simulink model "Model"  (R2022b)
settings: Solver=FixedStepAuto  StartTime=0.0  StopTime=ts  FixedStep=0.001  RelTol=1e-3
values from neighbouring files (symbols this model uses):
  A1 = 1    [Init.m]    (also in sh.m)
  A2 = 0    [Init.m]    (also in sh.m)
  alpha1 = 0.14    [Init.m]    (also in sh.m)
  alpha2 = 0    [Init.m]    (also in sh.m)
  base = 0.025    [Init.m]
  betta = 0    [Init.m]    (also in sh.m)
  ke = U/w    (= 0.690310596543)    [Init.m]
  km = i*(M/I)    (= 24.1911764706)    [Init.m]
  rad_wheel = 0.02    [Init.m]
  Tm = (J*w)/M0    (= 0.000140723404261)    [Init.m]
  x = 2    [Init.m]
  y = 2    [Init.m]    (also in Shum.m = block1+block2)
undefined symbols (not defined in the file or in its folder): out
libraries: simulink x3, fuzblock x1
settings Model: Creator=Адель  LastModifiedBy=Адель
settings ModelReferenceCC: EnableRefExpFcnMdlSchedulingChecks=on

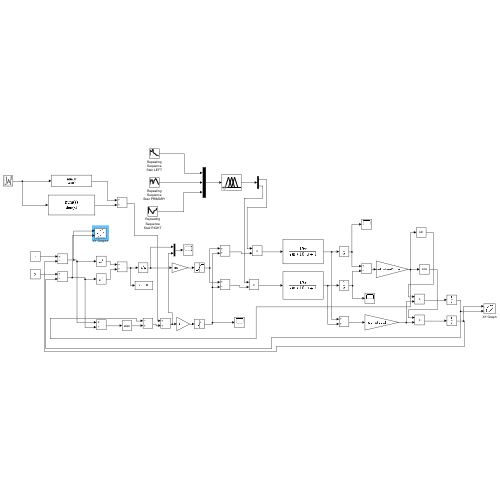
[thumbnail: Simulink's stored preview of the top-level diagram]
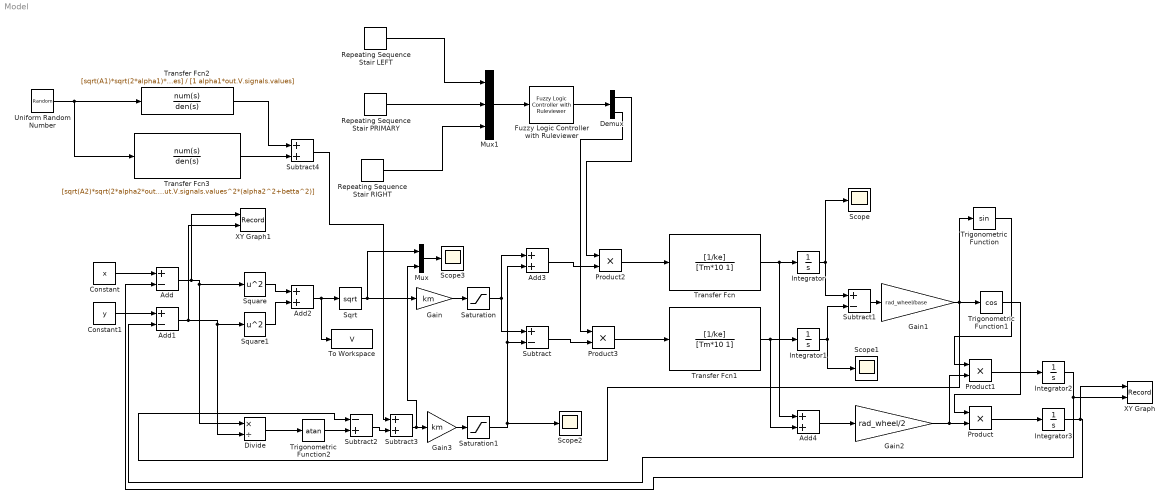
== system Model ==
  Add : Sum  Inputs=+-
  Add1 : Sum  Inputs=+-
  Add2 : Sum
  Add3 : Sum
  Add4 : Sum
  Constant : Constant  Value=x
  Constant1 : Constant  Value=y
  Demux : Demux  Outputs=2
  Divide : Product  Inputs=*/
  Fuzzy Logic Controller with Ruleviewer : fuzblock/Fuzzy Logic  Controller  with Ruleviewer  fismatrix=regulator  Ts=2
  Gain : Gain  Gain=km
  Gain1 : Gain  Gain=rad_wheel/base
  Gain2 : Gain  Gain=rad_wheel/2
  Gain3 : Gain  Gain=km
  Integrator{,1..3} (4 alike) : Integrator
  Mux : Mux  Inputs=2
  Mux1 : Mux  Inputs=3
  Product{,1..3} (4 alike) : Product
  Repeating Sequence Stair LEFT : simulink/Sources/Repeating Sequence Stair  OutValues=[35 33 40 27 25 22 19 18].'  tsamp=-1  OutMin=[]  OutMax=[]  OutDataTypeStr=double  OutputDataTypeScalingMode=double  OutDataType=fixdt(0,8)  ConRadixGroup=Best Precision: Vector-wise  OutScaling=2^-12
  Repeating Sequence Stair PRIMARY : simulink/Sources/Repeating Sequence Stair  OutValues=[35 33 40 41 42 33 22 26 39 40 45 50 47 42 36 31 24 16].'  tsamp=-1  OutMin=[]  OutMax=[]  OutDataTypeStr=double  OutputDataTypeScalingMode=double  OutDataType=fixdt(0,8)  ConRadixGroup=Best Precision: Vector-wise  OutScaling=2^-12
  Repeating Sequence Stair RIGHT : simulink/Sources/Repeating Sequence Stair  OutValues=[35 30 25 22 19 15 18 24 25 26 32].'  tsamp=-1  OutMin=[]  OutMax=[]  OutDataTypeStr=double  OutputDataTypeScalingMode=double  OutDataType=fixdt(0,8)  ConRadixGroup=Best Precision: Vector-wise  OutScaling=2^-12
  Saturation : Saturate  UpperLimit=5  LowerLimit=-5
  Saturation1 : Saturate  UpperLimit=5  LowerLimit=-5
  Scope{,1..3} (4 alike) : Scope
  Sqrt : Sqrt
  Square : Math  Operator=square
  Square1 : Math  Operator=square
  Subtract : Sum  Inputs=+-
  Subtract1 : Sum  Inputs=+-
  Subtract2 : Sum  Inputs=-+
  Subtract3 : Sum
  Subtract4 : Sum
  To Workspace : ToWorkspace  VariableName=V  SaveFormat=Structure  SampleTime=-1
      settings: MaxDataPoints=1  Save2DSignal=2-D array (concatenate along first dimension)
  Transfer Fcn : TransferFcn  Numerator=[1/ke]  Denominator=[Tm*10 1]
  Transfer Fcn1 : TransferFcn  Numerator=[1/ke]  Denominator=[Tm*10 1]
  Transfer Fcn2 : TransferFcn  Numerator=[sqrt(A1)*sqrt(2*alpha1)*out.V.signals.values]  Denominator=[1 alpha1*out.V.signals.values]
  Transfer Fcn3 : TransferFcn  Numerator=[sqrt(A2)*sqrt(2*alpha2*out.V.signals.values) out.V.signals.values*sqrt(A2)*sqrt(2*alpha2)*sqrt(alpha2^2+betta^2)]  Denominator=[1 alpha2 out.V.signals.values^2*(alpha2^2+betta^2)]
  Trigonometric Function : Trigonometry
  Trigonometric Function1 : Trigonometry  Operator=cos
  Trigonometric Function2 : Trigonometry  Operator=atan
  Uniform Random Number : UniformRandomNumber  SampleTime=0.1
  XY Graph : Record  FileSettingsInternal="{\"entries\":[{\"content\":{\"excelSettings\":{\"content\":{},\"type\":\"Streamout.ExcelSettings\"}},\"type\":\"Streamout.FileSettingStorage\",\"uuid\":\"aa12a716-93a2-48b4-a55e-da8b9cd06314\"}],\"packageUris\":[\"http://schema.mathworks.com/mf0/streamout_blocks/R2020a\"],\"version\":\"1.0\"}"  Layout=[1 1]  SignalsInternal="{\"entries\":[{\"content\":{\"signals\":[{\"content\":{\"blockPath\":[\"Model/XY Graph\"],\"channel\":[],\"dimensions\":[1],\"domain\":\"Model/XY Graph\",\"lineColor\":\"#a2142f\",\"plots\":[1],\"port\":1,\"sid\":[\"\"],\"signalID\":23953,\"signalName\":\"Integrator3\"},\"type\":\"RecordBlkView.Signal\",\"uuid\":\"0444dae7-0da9-414e-a023-1bf7262167d7\"},{\"content\":{\"blockPath\":[\"Model/XY Graph\"],\"channel\":[],\"dimensions\":[1],\"domain\":\"Model/XY Graph\",\"lineColor\":\"#139fff\",\"plots\":[1],\"port\":2,\"sid\":[\"\"],\"signalID\":23957,\"signalName\":\"Integrator2\"},\"type\":\"RecordBlkView.Signal\",\"uuid\":\"7eb82e51-9f61-4b1b-84a8-e7a589c59203\"}]},\"type\":\"RecordBlkView.InputSignals\",\"uuid\":\"91fa2a17-e54b-4373-83e1-be05bb8ce857\"}],\"packageUris\":[\"http://schema.mathworks.com/mf0/streamout_blocks/R2020a\"],\"version\":\"1.0\"}"  VisualizationBindings="{\"xyplotplugin\":{\"info\":[{\"series\":[{\"bindingParametersList\":[{\"parameter\":\"X-Axis\",\"signalID\":23953,\"signalName\":\"Integrator3\"},{\"parameter\":\"Y-Axis\",\"signalID\":23957,\"signalName\":\"Integrator2\"}],\"seriesID\":30355}],\"subplotID\":1}]}}"  CompatibilityTag=XY
  XY Graph1 : Record  FileSettingsInternal="{\"entries\":[{\"content\":{\"excelSettings\":{\"content\":{},\"type\":\"Streamout.ExcelSettings\"}},\"type\":\"Streamout.FileSettingStorage\",\"uuid\":\"9ece608a-e883-48e9-9140-3a9e7ef14128\"}],\"packageUris\":[\"http://schema.mathworks.com/mf0/streamout_blocks/R2020a\"],\"version\":\"1.0\"}"  Layout=[1 1]  SignalsInternal="{\"entries\":[{\"content\":{\"signals\":[{\"content\":{\"blockPath\":[\"Model/XY Graph1\"],\"channel\":[],\"dimensions\":[1],\"domain\":\"Model/XY Graph1\",\"lineColor\":\"#a2142f\",\"plots\":[1],\"port\":1,\"sid\":[\"\"],\"signalID\":23961,\"signalName\":\"Add\"},\"type\":\"RecordBlkView.Signal\",\"uuid\":\"d6554a96-d76f-4e85-b7c2-258af4738fcc\"},{\"content\":{\"blockPath\":[\"Model/XY Graph1\"],\"channel\":[],\"dimensions\":[1],\"domain\":\"Model/XY Graph1\",\"lineColor\":\"#139fff\",\"plots\":[1],\"port\":2,\"sid\":[\"\"],\"signalID\":23965,\"signalName\":\"Add1\"},\"type\":\"RecordBlkView.Signal\",\"uuid\":\"315f70b7-57a9-4ce5-8146-a3161a59c4c0\"}]},\"type\":\"RecordBlkView.InputSignals\",\"uuid\":\"67c831cd-9479-452f-ba01-f8b2655fe9d1\"}],\"packageUris\":[\"http://schema.mathworks.com/mf0/streamout_blocks/R2020a\"],\"version\":\"1.0\"}"  VisualizationBindings="{\"xyplotplugin\":{\"info\":[{\"series\":[{\"bindingParametersList\":[{\"parameter\":\"X-Axis\",\"signalID\":23961,\"signalName\":\"Add\"},{\"parameter\":\"Y-Axis\",\"signalID\":23965,\"signalName\":\"Add1\"}],\"seriesID\":54777}],\"subplotID\":1}]}}"  CompatibilityTag=XY
  wires:
  Constant/1 -> Add/1
  Constant1/1 -> Add1/1
  Add/1 -> XY Graph1/1, Divide/1, Square/1
  Add1/1 -> XY Graph1/2, Divide/2, Square1/1
  Square1/1 -> Add2/2
  Square/1 -> Add2/1
  Add2/1 -> To Workspace/1, Sqrt/1
  Gain/1 -> Saturation/1
  Saturation/1 -> Add3/1, Subtract/1
  Transfer Fcn/1 -> Add4/1, Integrator/1
  Transfer Fcn1/1 -> Add4/2, Integrator1/1
  Integrator/1 -> Scope/1, Subtract1/1
  Integrator1/1 -> Scope1/1, Subtract1/2
  Subtract1/1 -> Gain1/1
  Gain1/1 -> Trigonometric Function/1, Subtract2/1, Trigonometric Function1/1
  Add4/1 -> Gain2/1
  Gain2/1 -> Product1/2, Product/2
  Trigonometric Function1/1 -> Product/1
  Trigonometric Function/1 -> Product1/1
  Product1/1 -> Integrator2/1
  Product/1 -> Integrator3/1
  Integrator3/1 -> XY Graph/1, Add/2
  Integrator2/1 -> XY Graph/2, Add1/2
  Divide/1 -> Trigonometric Function2/1
  Trigonometric Function2/1 -> Subtract2/2
  Gain3/1 -> Saturation1/1
  Saturation1/1 -> Add3/2, Subtract/2, Scope2/1
  Mux/1 -> Scope3/1
  Subtract3/1 -> Mux/2, Gain3/1
  Subtract2/1 -> Subtract3/2
  Sqrt/1 -> Gain/1, Mux/1
  Transfer Fcn2/1 -> Subtract4/1
  Transfer Fcn3/1 -> Subtract4/2
  Uniform Random Number/1 -> Transfer Fcn2/1, Transfer Fcn3/1
  Subtract4/1 -> Subtract3/1
  Repeating Sequence Stair LEFT/1 -> Mux1/1
  Repeating Sequence Stair PRIMARY/1 -> Mux1/2
  Repeating Sequence Stair RIGHT/1 -> Mux1/3
  Fuzzy Logic Controller with Ruleviewer/1 -> Demux/1
  Mux1/1 -> Fuzzy Logic Controller with Ruleviewer/1
  Demux/1 -> Product2/1
  Demux/2 -> Product3/1
  Product2/1 -> Transfer Fcn/1
  Add3/1 -> Product2/2
  Product3/1 -> Transfer Fcn1/1
  Subtract/1 -> Product3/2
